simulink model "sistema"  (R2023a)
settings: Solver=ode23t  StartTime=0.0  StopTime=10  MaxStep=1E-3  RelTol=1e-3
libraries: fl_lib x21, nesl_utility x9, slpidlib x2
settings Model: LastModifiedBy=Kami Valle
settings DataIOCC: ReturnWorkspaceOutputs=off  TimeSaveName=t
settings DebuggingCC: AlgebraicLoopMsg=none  ArtificialAlgebraicLoopMsg=none  MaxConsecutiveZCsMsg=none
settings RTWCC: GPUComputeCapability=5.0

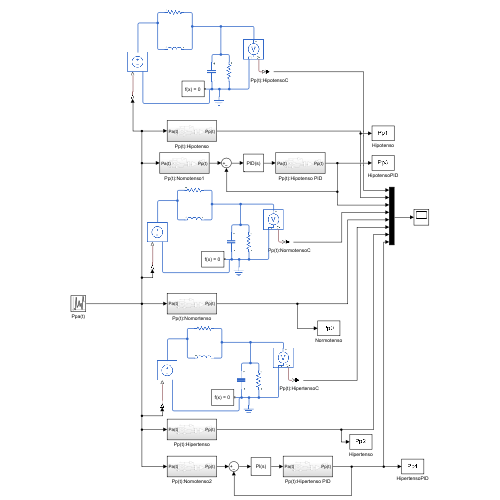
[thumbnail: Simulink's stored preview of the top-level diagram]
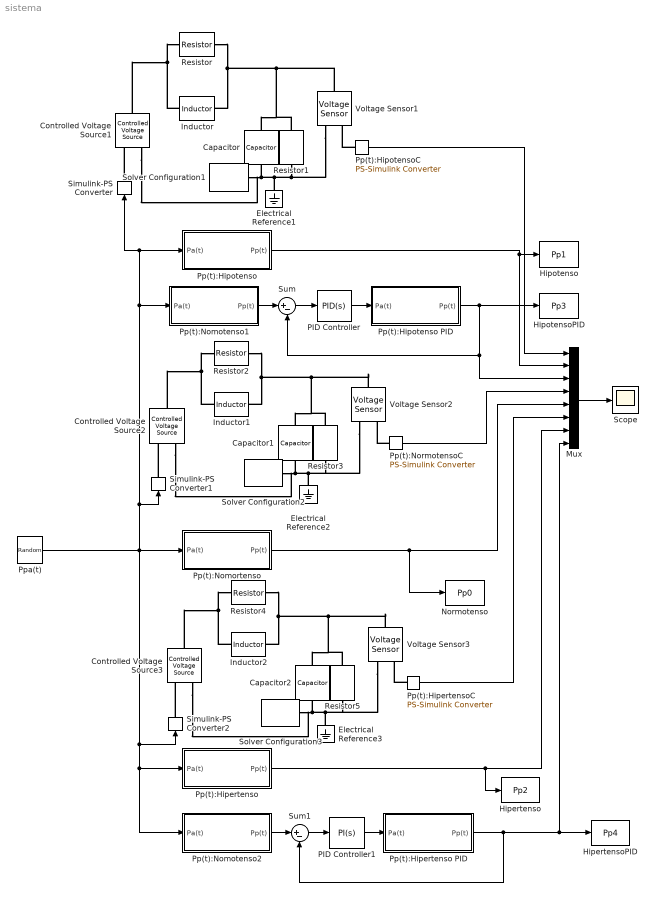
== system sistema ==
  Capacitor : fl_lib/Electrical/Electrical Elements/Capacitor  c=0.250 F  r=1e-6 Ohm  g=0 1/Ohm  i_specify=off  i_priority=None  i=0 A  i_nominal_specify=off  i_nominal_unit=A  i_nominal_value=1  v_specify=off  v_priority=None  v=0 V  v_nominal_specify=off  v_nominal_unit=V  v_nominal_value=1  vc_specify=off  vc_priority=High  vc=0 V  vc_nominal_specify=off  vc_nominal_unit=V  vc_nominal_value=1
  Capacitor1 : fl_lib/Electrical/Electrical Elements/Capacitor  c=1.500 F  r=1e-6 Ohm  g=0 1/Ohm  i_specify=off  i_priority=None  i=0 A  i_nominal_specify=off  i_nominal_unit=A  i_nominal_value=1  v_specify=off  v_priority=None  v=0 V  v_nominal_specify=off  v_nominal_unit=V  v_nominal_value=1  vc_specify=off  vc_priority=High  vc=0 V  vc_nominal_specify=off  vc_nominal_unit=V  vc_nominal_value=1
  Capacitor2 : fl_lib/Electrical/Electrical Elements/Capacitor  c=2.500 F  r=1e-6 Ohm  g=0 1/Ohm  i_specify=off  i_priority=None  i=0 A  i_nominal_specify=off  i_nominal_unit=A  i_nominal_value=1  v_specify=off  v_priority=None  v=0 V  v_nominal_specify=off  v_nominal_unit=V  v_nominal_value=1  vc_specify=off  vc_priority=High  vc=0 V  vc_nominal_specify=off  vc_nominal_unit=V  vc_nominal_value=1
  Controlled Voltage Source1 : fl_lib/Electrical/Electrical Sources/Controlled Voltage Source
  Controlled Voltage Source2 : fl_lib/Electrical/Electrical Sources/Controlled Voltage Source
  Controlled Voltage Source3 : fl_lib/Electrical/Electrical Sources/Controlled Voltage Source
  Electrical Reference1 : fl_lib/Electrical/Electrical Elements/Electrical Reference
  Electrical Reference2 : fl_lib/Electrical/Electrical Elements/Electrical Reference
  Electrical Reference3 : fl_lib/Electrical/Electrical Elements/Electrical Reference
  Hipertenso : ToWorkspace  VariableName=Pp2  SampleTime=-1
  HipertensoPID : ToWorkspace  VariableName=Pp4  SampleTime=-1
  Hipotenso : ToWorkspace  VariableName=Pp1  SampleTime=-1
  HipotensoPID : ToWorkspace  VariableName=Pp3  SampleTime=-1
  Inductor : fl_lib/Electrical/Electrical Elements/Inductor  l=0.005 H  r=0 Ohm  g=1e-9 1/Ohm  i_specify=off  i_priority=None  i=0 A  i_nominal_specify=off  i_nominal_unit=A  i_nominal_value=1  v_specify=off  v_priority=None  v=0 V  v_nominal_specify=off  v_nominal_unit=V  v_nominal_value=1  i_L_specify=off  i_L_priority=High  i_L=0 A  i_L_nominal_specify=off  i_L_nominal_unit=A  i_L_nominal_value=1
  Inductor1 : fl_lib/Electrical/Electrical Elements/Inductor  l=0.010 H  r=0 Ohm  g=1e-9 1/Ohm  i_specify=off  i_priority=None  i=0 A  i_nominal_specify=off  i_nominal_unit=A  i_nominal_value=1  v_specify=off  v_priority=None  v=0 V  v_nominal_specify=off  v_nominal_unit=V  v_nominal_value=1  i_L_specify=off  i_L_priority=High  i_L=0 A  i_L_nominal_specify=off  i_L_nominal_unit=A  i_L_nominal_value=1
  Inductor2 : fl_lib/Electrical/Electrical Elements/Inductor  l=0.020 H  r=0 Ohm  g=1e-9 1/Ohm  i_specify=off  i_priority=None  i=0 A  i_nominal_specify=off  i_nominal_unit=A  i_nominal_value=1  v_specify=off  v_priority=None  v=0 V  v_nominal_specify=off  v_nominal_unit=V  v_nominal_value=1  i_L_specify=off  i_L_priority=High  i_L=0 A  i_L_nominal_specify=off  i_L_nominal_unit=A  i_L_nominal_value=1
  Mux : Mux  Inputs=8
  Normotenso : ToWorkspace  VariableName=Pp0  SampleTime=-1
  PID Controller : slpidlib/PID Controller  Controller=PID  Form=Parallel  TimeDomain=Continuous-time  UseExternalTs=off  SampleTime=-1  IntegratorMethod=Forward Euler  FilterMethod=Forward Euler  ControllerParametersSource=internal  P=4.2164e-05  I=3267.6867  UseKiTs=off  D=0  N=100  UseFilter=on  TunerSelectOption=Transfer Function Based (PID Tuner App)  InitialConditionSource=internal  InitialConditionForIntegrator=0  InitialConditionForFilter=0  DifferentiatorICPrevScaledInput=0  ExternalReset=none  TrackingMode=off  Kt=1  LimitOutput=off  SatLimitsSource=internal  UpperSaturationLimit=inf  LowerSaturationLimit=-inf  LinearizeAsGain=on  AntiWindupMode=none  Kb=1  LimitIntegrator=off  UpperIntegratorSaturationLimit=inf  LowerIntegratorSaturationLimit=-inf  POutMin=[]  POutMax=[]  IOutMin=[]  IOutMax=[]  DOutMin=[]  DOutMax=[]  NOutMin=[]  NOutMax=[]  SumOutMin=[]  SumOutMax=[]  SaturationOutMin=[]  SaturationOutMax=[]  PParamMin=[]  PParamMax=[]  IParamMin=[]  IParamMax=[]  DParamMin=[]  DParamMax=[]  NParamMin=[]  NParamMax=[]  KbParamMin=[]  KbParamMax=[]  KtParamMin=[]  KtParamMax=[]  KbOutMin=[]  KbOutMax=[]  KtOutMin=[]  KtOutMax=[]  IntegratorOutMin=[]  IntegratorOutMax=[]  FilterOutMin=[]  FilterOutMax=[]  SumI1OutMin=[]  SumI1OutMax=[]  SumI2OutMin=[]  SumI2OutMax=[]  SumI3OutMin=[]  SumI3OutMax=[]  SumI4OutMin=[]  SumI4OutMax=[]  SumDOutMin=[]  SumDOutMax=[]  DifferentiatorOutMin=[]  DifferentiatorOutMax=[]  FilterDiffOutCoefMin=[]  FilterDiffOutCoefMax=[]  ReciprocalOutMin=[]  ReciprocalOutMax=[]  SumDenOutMin=[]  SumDenOutMax=[]  SumNumOutMin=[]  SumNumOutMax=[]  DivideOutMin=[]  DivideOutMax=[]  UdiffTsProdOutMin=[]  UdiffTsProdOutMax=[]  NTsProdOutMin=[]  NTsProdOutMax=[]  UintegralTsProdOutMin=[]  UintegralTsProdOutMax=[]  UngainTsProdOutMin=[]  UngainTsProdOutMax=[]  ClampingZeroOutDataTypeStr=Inherit: Inherit via back propagation  ClampingZeroOutMin=[]  ClampingZeroOutMax=[]  FilterDenConstantOutDataTypeStr=Inherit: Inherit via back propagation  FilterDenConstantOutMin=[]  FilterDenConstantOutMax=[]  PCopyOutDataTypeStr=Inherit: Inherit via back propagation  PCopyOutMin=[]  PCopyOutMax=[]  NCopyOutDataTypeStr=Inherit: Inherit via back propagation  NCopyOutMin=[]  NCopyOutMax=[]  IntegratorContinuousStateAttributes=''  IntegratorStateMustResolveToSignalObject=off  IntegratorRTWStateStorageClass=Auto  FilterContinuousStateAttributes=''  FilterStateMustResolveToSignalObject=off  FilterRTWStateStorageClass=Auto  ParallelPVariant=InternalParameters  IdealPVariant=Disabled  IVariant=InternalParameters  DVariant=InternalParameters  IntegratorVariant=Continuous  SatVariant=Disabled  AWVariant=Passthrough  PCopyVariant=Disabled  TRVariant=Disabled  FdbkBlocksVariant=Forward  IdealPFdbkVariant=Disabled  SatFdbkVariant=Disabled  DerivativeFilterVariant=ContFilter  NVariant=InternalParameters  NCopyVariant=Disabled  FilterICVariant=InternalICsFilter  IntegratorICVariant=InternalICs  ExternalResetVariant=Disabled  TRSumVariant=Passthrough  SumFdbkVariant=Disabled  SumVariant=Sum_PID  TsampFilterVariant=InternalTs  TsampNgainVariant=Passthrough  TsampIntegralVariant=Disabled_SignalSpec  ExternalSaturationOutDataTypeStr=Inherit: Same as second input
  PID Controller1 : slpidlib/PID Controller  Controller=PI  Form=Parallel  TimeDomain=Continuous-time  UseExternalTs=off  SampleTime=-1  IntegratorMethod=Forward Euler  FilterMethod=Forward Euler  ControllerParametersSource=internal  P=10  I=3275.21614803153  UseKiTs=off  D=1  N=1  UseFilter=on  TunerSelectOption=Transfer Function Based (PID Tuner App)  InitialConditionSource=internal  InitialConditionForIntegrator=0  InitialConditionForFilter=0  DifferentiatorICPrevScaledInput=0  ExternalReset=none  TrackingMode=off  Kt=1  LimitOutput=off  SatLimitsSource=internal  UpperSaturationLimit=inf  LowerSaturationLimit=-inf  LinearizeAsGain=on  AntiWindupMode=none  Kb=1  LimitIntegrator=off  UpperIntegratorSaturationLimit=inf  LowerIntegratorSaturationLimit=-inf  POutMin=[]  POutMax=[]  IOutMin=[]  IOutMax=[]  DOutMin=[]  DOutMax=[]  NOutMin=[]  NOutMax=[]  SumOutMin=[]  SumOutMax=[]  SaturationOutMin=[]  SaturationOutMax=[]  PParamMin=[]  PParamMax=[]  IParamMin=[]  IParamMax=[]  DParamMin=[]  DParamMax=[]  NParamMin=[]  NParamMax=[]  KbParamMin=[]  KbParamMax=[]  KtParamMin=[]  KtParamMax=[]  KbOutMin=[]  KbOutMax=[]  KtOutMin=[]  KtOutMax=[]  IntegratorOutMin=[]  IntegratorOutMax=[]  FilterOutMin=[]  FilterOutMax=[]  SumI1OutMin=[]  SumI1OutMax=[]  SumI2OutMin=[]  SumI2OutMax=[]  SumI3OutMin=[]  SumI3OutMax=[]  SumI4OutMin=[]  SumI4OutMax=[]  SumDOutMin=[]  SumDOutMax=[]  DifferentiatorOutMin=[]  DifferentiatorOutMax=[]  FilterDiffOutCoefMin=[]  FilterDiffOutCoefMax=[]  ReciprocalOutMin=[]  ReciprocalOutMax=[]  SumDenOutMin=[]  SumDenOutMax=[]  SumNumOutMin=[]  SumNumOutMax=[]  DivideOutMin=[]  DivideOutMax=[]  UdiffTsProdOutMin=[]  UdiffTsProdOutMax=[]  NTsProdOutMin=[]  NTsProdOutMax=[]  UintegralTsProdOutMin=[]  UintegralTsProdOutMax=[]  UngainTsProdOutMin=[]  UngainTsProdOutMax=[]  ClampingZeroOutDataTypeStr=Inherit: Inherit via back propagation  ClampingZeroOutMin=[]  ClampingZeroOutMax=[]  FilterDenConstantOutDataTypeStr=Inherit: Inherit via back propagation  FilterDenConstantOutMin=[]  FilterDenConstantOutMax=[]  PCopyOutDataTypeStr=Inherit: Inherit via back propagation  PCopyOutMin=[]  PCopyOutMax=[]  NCopyOutDataTypeStr=Inherit: Inherit via back propagation  NCopyOutMin=[]  NCopyOutMax=[]  IntegratorContinuousStateAttributes=''  IntegratorStateMustResolveToSignalObject=off  IntegratorRTWStateStorageClass=Auto  FilterContinuousStateAttributes=''  FilterStateMustResolveToSignalObject=off  FilterRTWStateStorageClass=Auto  ParallelPVariant=InternalParameters  IdealPVariant=Disabled  IVariant=InternalParameters  DVariant=Disabled  IntegratorVariant=Continuous  SatVariant=Disabled  AWVariant=Passthrough  PCopyVariant=Disabled  TRVariant=Disabled  FdbkBlocksVariant=Forward  IdealPFdbkVariant=Disabled  SatFdbkVariant=Disabled  DerivativeFilterVariant=Disabled  NVariant=Disabled  NCopyVariant=Disabled_SignalSpec  FilterICVariant=Disabled  IntegratorICVariant=InternalICs  ExternalResetVariant=Disabled  TRSumVariant=Passthrough  SumFdbkVariant=Disabled  SumVariant=Sum_PI  TsampFilterVariant=InternalTs  TsampNgainVariant=Passthrough  TsampIntegralVariant=Disabled_SignalSpec  ExternalSaturationOutDataTypeStr=Inherit: Same as second input
  Pp(t):Hipertenso : Subsystem
  Pp(t):Hipertenso PID : Subsystem
  Pp(t):HipertensoC : nesl_utility/PS-Simulink Converter  PhysicalDomain=network_engine_domain  SubClassName=ps_output  LeftPortType=input  RightPortType=output  PseudoPeriodic=off  Frequencies=[]  VectorFormat=1-D array  Unit=inherit  AffineConversion=off
  Pp(t):Hipotenso : Subsystem
  Pp(t):Hipotenso PID : Subsystem
  Pp(t):HipotensoC : nesl_utility/PS-Simulink Converter  PhysicalDomain=network_engine_domain  SubClassName=ps_output  LeftPortType=input  RightPortType=output  PseudoPeriodic=off  Frequencies=[]  VectorFormat=1-D array  Unit=inherit  AffineConversion=off
  Pp(t):Nomortenso : Subsystem
  Pp(t):Nomotenso1 : Subsystem
  Pp(t):Nomotenso2 : Subsystem
  Pp(t):NormotensoC : nesl_utility/PS-Simulink Converter  PhysicalDomain=network_engine_domain  SubClassName=ps_output  LeftPortType=input  RightPortType=output  PseudoPeriodic=off  Frequencies=[]  VectorFormat=1-D array  Unit=inherit  AffineConversion=off
  Ppa(t) : UniformRandomNumber  Minimum=-0.2  Seed=106  SampleTime=0.5
  Resistor : fl_lib/Electrical/Electrical Elements/Resistor  R=0.020 Ohm  i_specify=off  i_priority=None  i=0 A  i_nominal_specify=off  i_nominal_unit=A  i_nominal_value=1  v_specify=off  v_priority=None  v=0 V  v_nominal_specify=off  v_nominal_unit=V  v_nominal_value=1
  Resistor1 : fl_lib/Electrical/Electrical Elements/Resistor  R=0.600 Ohm  i_specify=off  i_priority=None  i=0 A  i_nominal_specify=off  i_nominal_unit=A  i_nominal_value=1  v_specify=off  v_priority=None  v=0 V  v_nominal_specify=off  v_nominal_unit=V  v_nominal_value=1
  Resistor2 : fl_lib/Electrical/Electrical Elements/Resistor  R=0.033 Ohm  i_specify=off  i_priority=None  i=0 A  i_nominal_specify=off  i_nominal_unit=A  i_nominal_value=1  v_specify=off  v_priority=None  v=0 V  v_nominal_specify=off  v_nominal_unit=V  v_nominal_value=1
  Resistor3 : fl_lib/Electrical/Electrical Elements/Resistor  R=0.950 Ohm  i_specify=off  i_priority=None  i=0 A  i_nominal_specify=off  i_nominal_unit=A  i_nominal_value=1  v_specify=off  v_priority=None  v=0 V  v_nominal_specify=off  v_nominal_unit=V  v_nominal_value=1
  Resistor4 : fl_lib/Electrical/Electrical Elements/Resistor  R=0.050 Ohm  i_specify=off  i_priority=None  i=0 A  i_nominal_specify=off  i_nominal_unit=A  i_nominal_value=1  v_specify=off  v_priority=None  v=0 V  v_nominal_specify=off  v_nominal_unit=V  v_nominal_value=1
  Resistor5 : fl_lib/Electrical/Electrical Elements/Resistor  R=1.400 Ohm  i_specify=off  i_priority=None  i=0 A  i_nominal_specify=off  i_nominal_unit=A  i_nominal_value=1  v_specify=off  v_priority=None  v=0 V  v_nominal_specify=off  v_nominal_unit=V  v_nominal_value=1
  Scope : Scope
  Simulink-PS Converter : nesl_utility/Simulink-PS Converter  PhysicalDomain=network_engine_domain  SubClassName=ps_input  LeftPortType=input  RightPortType=output  PseudoPeriodic=off  Frequencies=[]  NoiseDistribution=none  NoiseParameters=[]  Unit=1  AffineConversion=off  FilteringAndDerivatives=provide  SimscapeFilterOrder=1  InputFilterTimeConstant=0.001  UdotUserProvided=0
  Simulink-PS Converter1 : nesl_utility/Simulink-PS Converter  PhysicalDomain=network_engine_domain  SubClassName=ps_input  LeftPortType=input  RightPortType=output  PseudoPeriodic=off  Frequencies=[]  NoiseDistribution=none  NoiseParameters=[]  Unit=1  AffineConversion=off  FilteringAndDerivatives=provide  SimscapeFilterOrder=1  InputFilterTimeConstant=0.001  UdotUserProvided=0
  Simulink-PS Converter2 : nesl_utility/Simulink-PS Converter  PhysicalDomain=network_engine_domain  SubClassName=ps_input  LeftPortType=input  RightPortType=output  PseudoPeriodic=off  Frequencies=[]  NoiseDistribution=none  NoiseParameters=[]  Unit=1  AffineConversion=off  FilteringAndDerivatives=provide  SimscapeFilterOrder=1  InputFilterTimeConstant=0.001  UdotUserProvided=0
  Solver Configuration1 : nesl_utility/Solver Configuration  PhysicalDomain=network_engine_domain  SubClassName=solver  LeftPortType=input  RightPortType=generic  Tones=[]  Harmonics=[]  SimulateNoise=off  Profile=off  UseLocalSampling=off  EnableSwitchedLinearOptims=on  FrequencyDomain=off  UseCCode=off  RelTol=0.001  AbsTol=0.001  MinStep=1e-09  ToWorkspace=off  RevertToSquareIcSolve=off  NumHomotopyIterations=100  PhasorMode=off  PhasorModeNumHarmonics=1  ConsistencySolver=NEWTON_XTOL_AFTER_FTOL  IndexReductionMethod=DerivativeReplacement  DoDC=off  ResidualTolerance=1e-09  ConsistencyTolSource=GLOBAL  ConsistencyAbsTol=0.001  ConsistencyRelTol=0.001  ConsistencyTolFactor=0.001  UseLocalSolver=off  LocalSolverChoice=NE_BACKWARD_EULER_ADVANCER  ResolveIndetEquations=on  FunctionEvalNumThread=1  LocalSolverSampleTime=0.001  DoFixedCost=off  MaxNonlinIter=3  MaxModeIter=2  ComputeImpulses=off  ImpulseIterations=2  LinearAlgebra=auto  LinearAlgebraNumThread=0  EquationFormulation=NE_TIME_EF  DelaysMemoryBudget=1024  AutomaticFiltering=on  FilteringTimeConstant=0.001  PartitionStorageMethod=AS_NEEDED  PartitionMemoryBudget=1024  PartitionMethod=ROBUST
  Solver Configuration2 : nesl_utility/Solver Configuration  PhysicalDomain=network_engine_domain  SubClassName=solver  LeftPortType=input  RightPortType=generic  Tones=[]  Harmonics=[]  SimulateNoise=off  Profile=off  UseLocalSampling=off  EnableSwitchedLinearOptims=on  FrequencyDomain=off  UseCCode=off  RelTol=0.001  AbsTol=0.001  MinStep=1e-09  ToWorkspace=off  RevertToSquareIcSolve=off  NumHomotopyIterations=100  PhasorMode=off  PhasorModeNumHarmonics=1  ConsistencySolver=NEWTON_XTOL_AFTER_FTOL  IndexReductionMethod=DerivativeReplacement  DoDC=off  ResidualTolerance=1e-09  ConsistencyTolSource=GLOBAL  ConsistencyAbsTol=0.001  ConsistencyRelTol=0.001  ConsistencyTolFactor=0.001  UseLocalSolver=off  LocalSolverChoice=NE_BACKWARD_EULER_ADVANCER  ResolveIndetEquations=on  FunctionEvalNumThread=1  LocalSolverSampleTime=0.001  DoFixedCost=off  MaxNonlinIter=3  MaxModeIter=2  ComputeImpulses=off  ImpulseIterations=2  LinearAlgebra=auto  LinearAlgebraNumThread=0  EquationFormulation=NE_TIME_EF  DelaysMemoryBudget=1024  AutomaticFiltering=on  FilteringTimeConstant=0.001  PartitionStorageMethod=AS_NEEDED  PartitionMemoryBudget=1024  PartitionMethod=ROBUST
  Solver Configuration3 : nesl_utility/Solver Configuration  PhysicalDomain=network_engine_domain  SubClassName=solver  LeftPortType=input  RightPortType=generic  Tones=[]  Harmonics=[]  SimulateNoise=off  Profile=off  UseLocalSampling=off  EnableSwitchedLinearOptims=on  FrequencyDomain=off  UseCCode=off  RelTol=0.001  AbsTol=0.001  MinStep=1e-09  ToWorkspace=off  RevertToSquareIcSolve=off  NumHomotopyIterations=100  PhasorMode=off  PhasorModeNumHarmonics=1  ConsistencySolver=NEWTON_XTOL_AFTER_FTOL  IndexReductionMethod=DerivativeReplacement  DoDC=off  ResidualTolerance=1e-09  ConsistencyTolSource=GLOBAL  ConsistencyAbsTol=0.001  ConsistencyRelTol=0.001  ConsistencyTolFactor=0.001  UseLocalSolver=off  LocalSolverChoice=NE_BACKWARD_EULER_ADVANCER  ResolveIndetEquations=on  FunctionEvalNumThread=1  LocalSolverSampleTime=0.001  DoFixedCost=off  MaxNonlinIter=3  MaxModeIter=2  ComputeImpulses=off  ImpulseIterations=2  LinearAlgebra=auto  LinearAlgebraNumThread=0  EquationFormulation=NE_TIME_EF  DelaysMemoryBudget=1024  AutomaticFiltering=on  FilteringTimeConstant=0.001  PartitionStorageMethod=AS_NEEDED  PartitionMemoryBudget=1024  PartitionMethod=ROBUST
  Sum : Sum  Inputs=|+-
  Sum1 : Sum  Inputs=|+-
  Voltage Sensor1 : fl_lib/Electrical/Electrical Sensors/Voltage Sensor
  Voltage Sensor2 : fl_lib/Electrical/Electrical Sensors/Voltage Sensor
  Voltage Sensor3 : fl_lib/Electrical/Electrical Sensors/Voltage Sensor
  wires:
  Mux/1 -> Scope/1
  Pp(t):Nomortenso/1(Pp(t)) -> Normotenso/1, Mux/5
  Pp(t):HipotensoC/1 -> Mux/1
  Ppa(t)/1 -> Pp(t):Nomortenso/1(Pa(t)), Simulink-PS Converter2/1, Pp(t):Nomotenso2/1(Pa(t)), Pp(t):Hipertenso/1(Pa(t)), Simulink-PS Converter1/1, Pp(t):Nomotenso1/1(Pa(t)), Pp(t):Hipotenso/1(Pa(t)), Simulink-PS Converter/1
  Pp(t):Nomotenso1/1(Pp(t)) -> Sum/1
  Sum/1 -> PID Controller/1
  PID Controller/1 -> Pp(t):Hipotenso PID/1(Pa(t))
  Pp(t):Hipotenso PID/1(Pp(t)) -> Mux/3, Sum/2, HipotensoPID/1
  Pp(t):Nomotenso2/1(Pp(t)) -> Sum1/1
  Pp(t):Hipertenso PID/1(Pp(t)) -> Sum1/2, Mux/8, HipertensoPID/1
  Sum1/1 -> PID Controller1/1
  PID Controller1/1 -> Pp(t):Hipertenso PID/1(Pa(t))
  Pp(t):Hipotenso/1(Pp(t)) -> Hipotenso/1, Mux/2
  Pp(t):NormotensoC/1 -> Mux/4
  Pp(t):HipertensoC/1 -> Mux/6
  Pp(t):Hipertenso/1(Pp(t)) -> Hipertenso/1, Mux/7
  connections:
  Inductor/LConn1 -- Controlled Voltage Source1/LConn1 -- Resistor/LConn1
  Resistor/RConn1 -- Capacitor/LConn1 -- Resistor1/LConn1 -- Voltage Sensor1/LConn1 -- Inductor/RConn1
  Resistor1/RConn1 -- Voltage Sensor1/RConn2 -- Electrical Reference1/LConn1 -- Controlled Voltage Source1/RConn2 -- Solver Configuration1/RConn1 -- Capacitor/RConn1
  Simulink-PS Converter/RConn1 -- Controlled Voltage Source1/RConn1
  Pp(t):HipotensoC/LConn1 -- Voltage Sensor1/RConn1
  Resistor2/RConn1 -- Capacitor1/LConn1 -- Resistor3/LConn1 -- Voltage Sensor2/LConn1 -- Inductor1/RConn1
  Capacitor1/RConn1 -- Voltage Sensor2/RConn2 -- Resistor3/RConn1 -- Electrical Reference2/LConn1 -- Controlled Voltage Source2/RConn2 -- Solver Configuration2/RConn1
  Inductor1/LConn1 -- Controlled Voltage Source2/LConn1 -- Resistor2/LConn1
  Pp(t):NormotensoC/LConn1 -- Voltage Sensor2/RConn1
  Simulink-PS Converter1/RConn1 -- Controlled Voltage Source2/RConn1
  Capacitor2/RConn1 -- Controlled Voltage Source3/RConn2 -- Solver Configuration3/RConn1 -- Voltage Sensor3/RConn2 -- Resistor5/RConn1 -- Electrical Reference3/LConn1
  Resistor4/RConn1 -- Inductor2/RConn1 -- Voltage Sensor3/LConn1 -- Capacitor2/LConn1 -- Resistor5/LConn1
  Inductor2/LConn1 -- Controlled Voltage Source3/LConn1 -- Resistor4/LConn1
  Pp(t):HipertensoC/LConn1 -- Voltage Sensor3/RConn1
  Simulink-PS Converter2/RConn1 -- Controlled Voltage Source3/RConn1

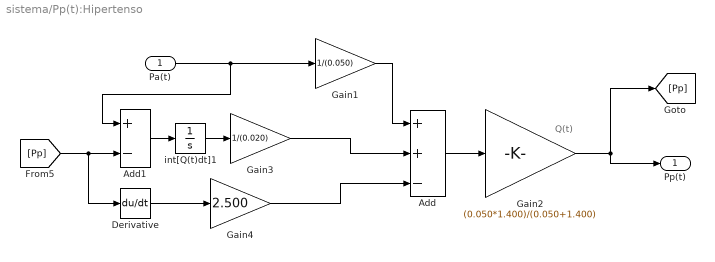
== system sistema/Pp(t):Hipertenso ==
  note: Q(t)
  Pa(t) : Inport
  Add : Sum  Inputs=++-
  Add1 : Sum  Inputs=+-
  Derivative : Derivative
  Gain1 : Gain  Gain=1/(0.050)
  Gain2 : Gain  Gain=(0.050*1.400)/(0.050+1.400)
  Gain3 : Gain  Gain=1/(0.020)
  Gain4 : Gain  Gain=2.500
  int[Q(t)dt]1 : Integrator
  Pp(t) : Outport
  wires:
  Add/1 -> Gain2/1
  Gain2/1 -> Pp(t)/1, [Pp]
  Pa(t)/1 -> Gain1/1, Add1/1
  Gain1/1 -> Add/1
  [Pp] -> Derivative/1, Add1/2
  Add1/1 -> int[Q(t)dt]1/1
  int[Q(t)dt]1/1 -> Gain3/1
  Gain3/1 -> Add/2
  Derivative/1 -> Gain4/1
  Gain4/1 -> Add/3

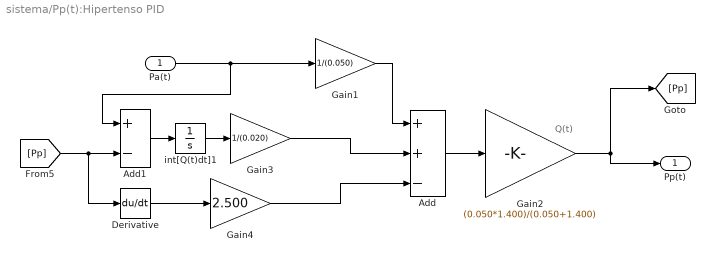
== system sistema/Pp(t):Hipertenso PID ==
  note: Q(t)
  Pa(t) : Inport
  Add : Sum  Inputs=++-
  Add1 : Sum  Inputs=+-
  Derivative : Derivative
  Gain1 : Gain  Gain=1/(0.050)
  Gain2 : Gain  Gain=(0.050*1.400)/(0.050+1.400)
  Gain3 : Gain  Gain=1/(0.020)
  Gain4 : Gain  Gain=2.500
  int[Q(t)dt]1 : Integrator
  Pp(t) : Outport
  wires:
  Add/1 -> Gain2/1
  Gain2/1 -> Pp(t)/1, [Pp]
  Pa(t)/1 -> Gain1/1, Add1/1
  Gain1/1 -> Add/1
  [Pp] -> Derivative/1, Add1/2
  Add1/1 -> int[Q(t)dt]1/1
  int[Q(t)dt]1/1 -> Gain3/1
  Gain3/1 -> Add/2
  Derivative/1 -> Gain4/1
  Gain4/1 -> Add/3

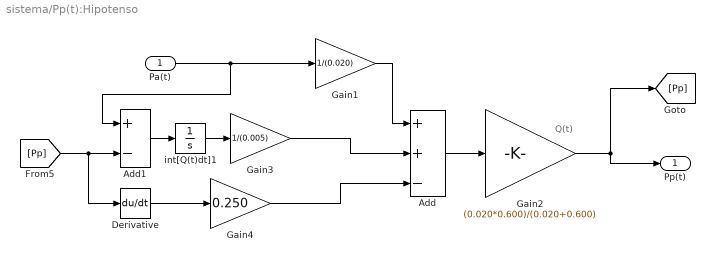
== system sistema/Pp(t):Hipotenso ==
  note: Q(t)
  Pa(t) : Inport
  Add : Sum  Inputs=++-
  Add1 : Sum  Inputs=+-
  Derivative : Derivative
  Gain1 : Gain  Gain=1/(0.020)
  Gain2 : Gain  Gain=(0.020*0.600)/(0.020+0.600)
  Gain3 : Gain  Gain=1/(0.005)
  Gain4 : Gain  Gain=0.250
  int[Q(t)dt]1 : Integrator
  Pp(t) : Outport
  wires:
  Add/1 -> Gain2/1
  Gain2/1 -> Pp(t)/1, [Pp]
  Pa(t)/1 -> Gain1/1, Add1/1
  Gain1/1 -> Add/1
  [Pp] -> Derivative/1, Add1/2
  Add1/1 -> int[Q(t)dt]1/1
  int[Q(t)dt]1/1 -> Gain3/1
  Gain3/1 -> Add/2
  Derivative/1 -> Gain4/1
  Gain4/1 -> Add/3

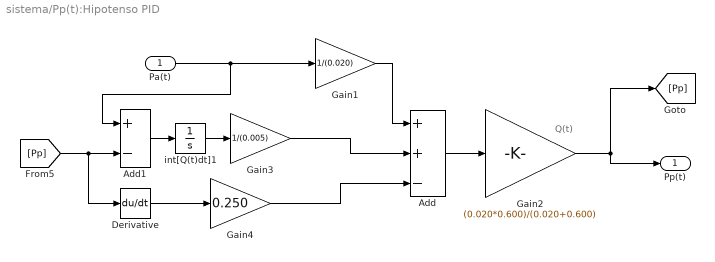
== system sistema/Pp(t):Hipotenso PID ==
  note: Q(t)
  Pa(t) : Inport
  Add : Sum  Inputs=++-
  Add1 : Sum  Inputs=+-
  Derivative : Derivative
  Gain1 : Gain  Gain=1/(0.020)
  Gain2 : Gain  Gain=(0.020*0.600)/(0.020+0.600)
  Gain3 : Gain  Gain=1/(0.005)
  Gain4 : Gain  Gain=0.250
  int[Q(t)dt]1 : Integrator
  Pp(t) : Outport
  wires:
  Add/1 -> Gain2/1
  Gain2/1 -> Pp(t)/1, [Pp]
  Pa(t)/1 -> Gain1/1, Add1/1
  Gain1/1 -> Add/1
  [Pp] -> Derivative/1, Add1/2
  Add1/1 -> int[Q(t)dt]1/1
  int[Q(t)dt]1/1 -> Gain3/1
  Gain3/1 -> Add/2
  Derivative/1 -> Gain4/1
  Gain4/1 -> Add/3

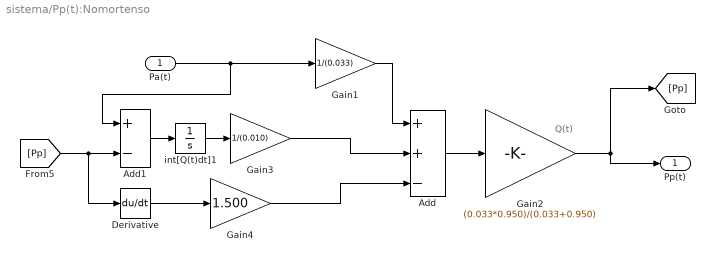
== system sistema/Pp(t):Nomortenso ==
  note: Q(t)
  Pa(t) : Inport
  Add : Sum  Inputs=++-
  Add1 : Sum  Inputs=+-
  Derivative : Derivative
  Gain1 : Gain  Gain=1/(0.033)
  Gain2 : Gain  Gain=(0.033*0.950)/(0.033+0.950)
  Gain3 : Gain  Gain=1/(0.010)
  Gain4 : Gain  Gain=1.500
  int[Q(t)dt]1 : Integrator
  Pp(t) : Outport
  wires:
  Add/1 -> Gain2/1
  Gain2/1 -> Pp(t)/1, [Pp]
  Pa(t)/1 -> Gain1/1, Add1/1
  Gain1/1 -> Add/1
  [Pp] -> Derivative/1, Add1/2
  Add1/1 -> int[Q(t)dt]1/1
  int[Q(t)dt]1/1 -> Gain3/1
  Gain3/1 -> Add/2
  Derivative/1 -> Gain4/1
  Gain4/1 -> Add/3

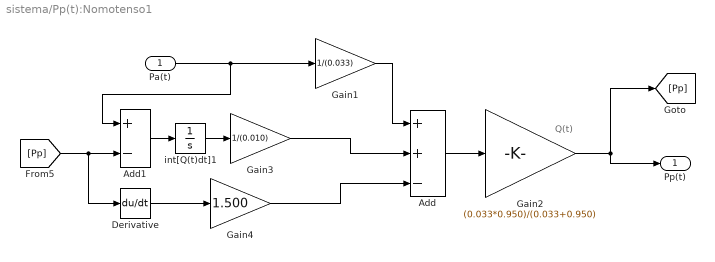
== system sistema/Pp(t):Nomotenso1 ==
  note: Q(t)
  Pa(t) : Inport
  Add : Sum  Inputs=++-
  Add1 : Sum  Inputs=+-
  Derivative : Derivative
  Gain1 : Gain  Gain=1/(0.033)
  Gain2 : Gain  Gain=(0.033*0.950)/(0.033+0.950)
  Gain3 : Gain  Gain=1/(0.010)
  Gain4 : Gain  Gain=1.500
  int[Q(t)dt]1 : Integrator
  Pp(t) : Outport
  wires:
  Add/1 -> Gain2/1
  Gain2/1 -> Pp(t)/1, [Pp]
  Pa(t)/1 -> Gain1/1, Add1/1
  Gain1/1 -> Add/1
  [Pp] -> Derivative/1, Add1/2
  Add1/1 -> int[Q(t)dt]1/1
  int[Q(t)dt]1/1 -> Gain3/1
  Gain3/1 -> Add/2
  Derivative/1 -> Gain4/1
  Gain4/1 -> Add/3

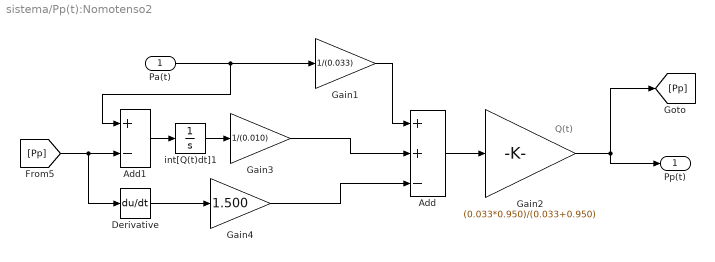
== system sistema/Pp(t):Nomotenso2 ==
  note: Q(t)
  Pa(t) : Inport
  Add : Sum  Inputs=++-
  Add1 : Sum  Inputs=+-
  Derivative : Derivative
  Gain1 : Gain  Gain=1/(0.033)
  Gain2 : Gain  Gain=(0.033*0.950)/(0.033+0.950)
  Gain3 : Gain  Gain=1/(0.010)
  Gain4 : Gain  Gain=1.500
  int[Q(t)dt]1 : Integrator
  Pp(t) : Outport
  wires:
  Add/1 -> Gain2/1
  Gain2/1 -> Pp(t)/1, [Pp]
  Pa(t)/1 -> Gain1/1, Add1/1
  Gain1/1 -> Add/1
  [Pp] -> Derivative/1, Add1/2
  Add1/1 -> int[Q(t)dt]1/1
  int[Q(t)dt]1/1 -> Gain3/1
  Gain3/1 -> Add/2
  Derivative/1 -> Gain4/1
  Gain4/1 -> Add/3
